simulink model "ControlOrientedModelsOfSeriesHybridElectricPowertrain"  (R2018b)
settings: Solver=VariableStepAuto  StartTime=0.0  StopTime=400  FixedStep=Tp  RelTol=1e-3
values from neighbouring files (symbols this model uses):
  R_wheel = 0.3    [data.mat]
  road =     [data.mat]
  StartPosition = 1600    [data.mat]
  V0 = 0    [data.mat]
undefined symbols (not defined in the file or in its folder): magnitude
libraries: simulink x6, simulink_extras x2, autolibshared x1
settings Model: SimulationMode=accelerator  Creator=piotr  LastModifiedBy=piotr
settings SolverCC: MaxConsecutiveMinStep=auto  ZeroCrossAlgorithm=Adaptive
settings OptimizationCC: EfficientMapNaN2IntZero=off
settings DebuggingCC: IgnoredZcDiagnostic=none  UnderSpecifiedDimensionMsg=warning
settings HardwareCC: TargetBitPerLong=64  TargetBitPerPointer=64  TargetBitPerSizeT=64  TargetBitPerPtrDiffT=64  TargetLongLongMode=on  TargetIntDivRoundTo=Zero  TargetEndianess=LittleEndian  TargetWordSize=64  TargetHWDeviceType=MATLAB Host  ProdEqTarget=off
settings CodeAppCC: MaxIdLength=128
settings GRTTargetCC: TargetLangStandard=C89/C90 (ANSI)  CombineOutputUpdateFcns=off  GRTInterface=on

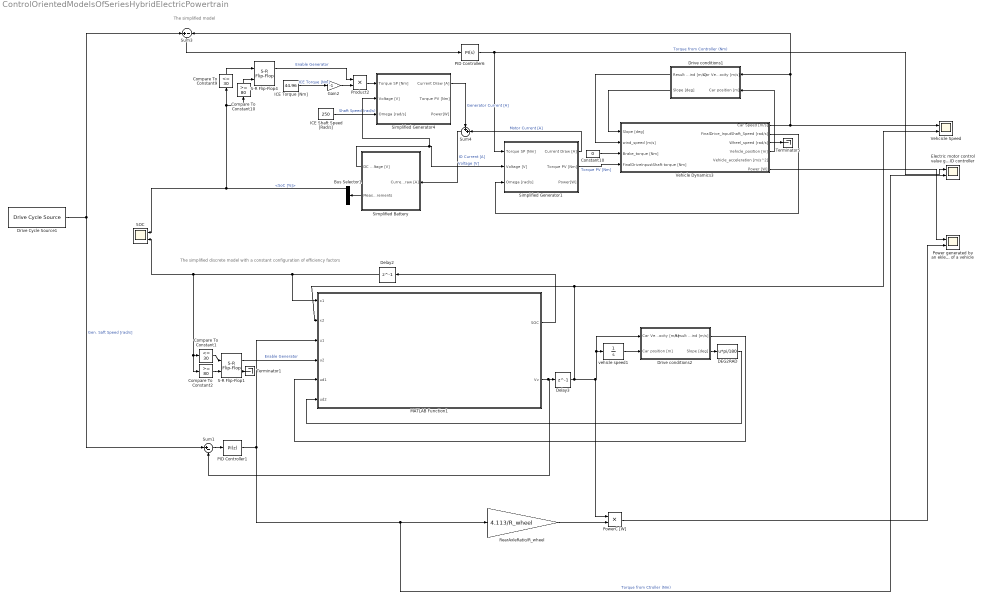
== system ControlOrientedModelsOfSeriesHybridElectricPowertrain ==
  note: The simplified discrete model with a constant configuration of efficiency factors
  note: The simplified model
  Bus Selector1 : BusSelector  OutputSignals=SoC [%],Power [W],IO Current [A]
  Compare To Constant1 : simulink/Logic and Bit Operations/Compare To Constant  relop=<=  const=30  OutDataTypeStr=boolean
  Compare To Constant10 : simulink/Logic and Bit Operations/Compare To Constant  relop=>=  const=80  OutDataTypeStr=boolean
  Compare To Constant2 : simulink/Logic and Bit Operations/Compare To Constant  relop=>=  const=80  OutDataTypeStr=boolean
  Compare To Constant9 : simulink/Logic and Bit Operations/Compare To Constant  relop=<=  const=30  OutDataTypeStr=boolean
  Constant10 : Constant  Value=0
  DEG2RAD : Fcn  Expr=u*pi/180
  Delay2 : Delay  DelayLength=1  InitialCondition=31  SampleTime=0.001
  Delay3 : Delay  DelayLength=1  InitialCondition=0  SampleTime=0.001
  Drive Cycle Source1 : autolibshared/Drive Cycle Source  cycleVar=FTP75  fileVar=cycleFTP75.mat  tfinal="2474  seconds"  cycleRepeat=off  outAccPort=off  outGearPort=off  gearList=No gear data  t_wot1=5  xdot_woto=0  xdot_wot1=30  t_wot2=20  xdot_wot2=0  t_wotend=30  srcUnit=m/s  outUnit=m/s  srcAccUnit=m/s/s  outAccUnit=m/s^2  dt=0  aMode=1
      settings: SourceProductName=Powertrain Blockset  SourceProductBaseCode=PW
  Drive conditions1 : Subsystem
  Drive conditions2 : Subsystem
  Electric motor control value generated by the PID controller : Scope  NumInputPorts=2
  Gain2 : Gain  Gain=-1
  ICE Shaft Speed [Rad/s] : Constant  Value=250
  ICE Torque [Nm] : Constant  Value=44.96
  MATLAB Function1 : MATLAB Function  TreatAsAtomicUnit=on
  PID Controller1 : simulink/Continuous/PID Controller  Controller=PI  Form=Parallel  TimeDomain=Discrete-time  SampleTime=0.001  IntegratorMethod=Forward Euler  FilterMethod=Forward Euler  ControllerParametersSource=internal  P=50  I=5  D=0  UseFilter=on  N=100  TunerSelectOption=Transfer Function Based (PID Tuner App)  InitialConditionSource=internal  InitialConditionForIntegrator=0  InitialConditionForFilter=0  DifferentiatorICPrevScaledInput=0  ExternalReset=none  TrackingMode=off  Kt=1  LimitOutput=off  UpperSaturationLimit=inf  LowerSaturationLimit=-inf  LinearizeAsGain=on  AntiWindupMode=none  Kb=1  POutMin=[]  POutMax=[]  IOutMin=[]  IOutMax=[]  DOutMin=[]  DOutMax=[]  NOutMin=[]  NOutMax=[]  SumOutMin=[]  SumOutMax=[]  SaturationOutMin=[]  SaturationOutMax=[]  PParamMin=[]  PParamMax=[]  IParamMin=[]  IParamMax=[]  DParamMin=[]  DParamMax=[]  NParamMin=[]  NParamMax=[]  KbParamMin=[]  KbParamMax=[]  KtParamMin=[]  KtParamMax=[]  KbOutMin=[]  KbOutMax=[]  KtOutMin=[]  KtOutMax=[]  IntegratorOutMin=[]  IntegratorOutMax=[]  FilterOutMin=[]  FilterOutMax=[]  SumI1OutMin=[]  SumI1OutMax=[]  SumI2OutMin=[]  SumI2OutMax=[]  SumI3OutMin=[]  SumI3OutMax=[]  SumI4OutMin=[]  SumI4OutMax=[]  SumDOutMin=[]  SumDOutMax=[]  DifferentiatorOutMin=[]  DifferentiatorOutMax=[]  FilterDiffOutCoefMin=[]  FilterDiffOutCoefMax=[]  ReciprocalOutMin=[]  ReciprocalOutMax=[]  SumDenOutMin=[]  SumDenOutMax=[]  SumNumOutMin=[]  SumNumOutMax=[]  DivideOutMin=[]  DivideOutMax=[]  IntegratorContinuousStateAttributes=''  IntegratorStateMustResolveToSignalObject=off  IntegratorRTWStateStorageClass=Auto  FilterContinuousStateAttributes=''  FilterStateMustResolveToSignalObject=off  FilterRTWStateStorageClass=Auto  ParallelPVariant=InternalParameters  IdealPVariant=Disabled  IVariant=InternalParameters  DVariant=Disabled  IntegratorVariant=Discrete  SatVariant=Disabled  AWVariant=Passthrough  PCopyVariant=Disabled  TRVariant=Disabled  FdbkBlocksVariant=Forward  IdealPFdbkVariant=Disabled  SatFdbkVariant=Disabled  DerivativeFilterVariant=Disabled  NVariant=Disabled  NCopyVariant=Disabled_SignalSpec  FilterICVariant=Disabled  IntegratorICVariant=InternalICs  ExternalResetVariant=Disabled  TRSumVariant=Passthrough  SumFdbkVariant=Disabled  SumVariant=Sum_PI
  PID Controller6 : simulink/Continuous/PID Controller  Controller=PI  Form=Parallel  TimeDomain=Continuous-time  SampleTime=-1  IntegratorMethod=Forward Euler  FilterMethod=Forward Euler  ControllerParametersSource=internal  P=50  I=5  D=0  UseFilter=on  N=100  TunerSelectOption=Transfer Function Based (PID Tuner App)  InitialConditionSource=internal  InitialConditionForIntegrator=0  InitialConditionForFilter=0  DifferentiatorICPrevScaledInput=0  ExternalReset=none  TrackingMode=off  Kt=1  LimitOutput=off  UpperSaturationLimit=inf  LowerSaturationLimit=-inf  LinearizeAsGain=on  AntiWindupMode=none  Kb=1  POutMin=[]  POutMax=[]  IOutMin=[]  IOutMax=[]  DOutMin=[]  DOutMax=[]  NOutMin=[]  NOutMax=[]  SumOutMin=[]  SumOutMax=[]  SaturationOutMin=[]  SaturationOutMax=[]  PParamMin=[]  PParamMax=[]  IParamMin=[]  IParamMax=[]  DParamMin=[]  DParamMax=[]  NParamMin=[]  NParamMax=[]  KbParamMin=[]  KbParamMax=[]  KtParamMin=[]  KtParamMax=[]  KbOutMin=[]  KbOutMax=[]  KtOutMin=[]  KtOutMax=[]  IntegratorOutMin=[]  IntegratorOutMax=[]  FilterOutMin=[]  FilterOutMax=[]  SumI1OutMin=[]  SumI1OutMax=[]  SumI2OutMin=[]  SumI2OutMax=[]  SumI3OutMin=[]  SumI3OutMax=[]  SumI4OutMin=[]  SumI4OutMax=[]  SumDOutMin=[]  SumDOutMax=[]  DifferentiatorOutMin=[]  DifferentiatorOutMax=[]  FilterDiffOutCoefMin=[]  FilterDiffOutCoefMax=[]  ReciprocalOutMin=[]  ReciprocalOutMax=[]  SumDenOutMin=[]  SumDenOutMax=[]  SumNumOutMin=[]  SumNumOutMax=[]  DivideOutMin=[]  DivideOutMax=[]  IntegratorContinuousStateAttributes=''  IntegratorStateMustResolveToSignalObject=off  IntegratorRTWStateStorageClass=Auto  FilterContinuousStateAttributes=''  FilterStateMustResolveToSignalObject=off  FilterRTWStateStorageClass=Auto  ParallelPVariant=InternalParameters  IdealPVariant=Disabled  IVariant=InternalParameters  DVariant=Disabled  IntegratorVariant=Continuous  SatVariant=Disabled  AWVariant=Passthrough  PCopyVariant=Disabled  TRVariant=Disabled  FdbkBlocksVariant=Forward  IdealPFdbkVariant=Disabled  SatFdbkVariant=Disabled  DerivativeFilterVariant=Disabled  NVariant=Disabled  NCopyVariant=Disabled_SignalSpec  FilterICVariant=Disabled  IntegratorICVariant=InternalICs  ExternalResetVariant=Disabled  TRSumVariant=Passthrough  SumFdbkVariant=Disabled  SumVariant=Sum_PI
  "Power generated by an eklectric motor driving the wheels of a vehicle " : Scope  NumInputPorts=2
  PowerC [W] : Product
  Product2 : Product
  RearAxleRatio/R_wheel : Gain  Gain=4.113/R_wheel
  S-R Flip-Flop1 : simulink_extras/Flip Flops/S-R Flip-Flop  initial_condition=0
  S-R Flip-Flop4 : simulink_extras/Flip Flops/S-R Flip-Flop  initial_condition=0
  "SOC " : Scope  NumInputPorts=2
  Simplified Battery : Subsystem  mask(Simple Battery with DC/DC converter){VIO=500, VBatt=200, CapBatt=7, Isoc=31, CHCoeff=75, DCoeff=90}
      mask prompts: VIO "DC Source Voltage I/O"; VBatt "DC Battery Inside Model Voltage"; CapBatt "Battery Capacity [Ah] Reffers to Battery Inside Model Voltage"; Isoc "Initial SOC [0-100%]"; CHCoeff "Charging Coefficient [0-100%]"; DCoeff "Draw Energy Coefficient [0-100%]"
  Simplified Generator1 : Subsystem  mask(Simplify Electric Motor/Generator){GCoeff=85, UCoeff=100}
      mask prompts: GCoeff "Generator performance [0-100%]"; UCoeff "Motor Performance [0-100%]"
      mask help: Block converts electric energy into mechanical energy. Torque set point is limited by torque vs speed table. Block calculates current draw and electric motor/generator torque within given radial speed. In Generator mode negative torque gives current.
  Simplified Generator4 : Subsystem  mask(Simplify Electric Motor/Generator){GCoeff=95, UCoeff=100}
      mask prompts: GCoeff "Generator performance [0-100%]"; UCoeff "Motor Performance [0-100%]"
      mask help: Block converts electric energy into mechanical energy. Torque set point is limited by torque vs speed table. Block calculates current draw and electric motor/generator torque within given radial speed. In Generator mode negative torque gives current.
  Sum1 : Sum  Inputs=|+-
  Sum3 : Sum  Inputs=+-
  Sum4 : Sum  Inputs=++|
  Terminator1 : Terminator
  Terminator5 : Terminator
  Vehcicle Speed : Scope  NumInputPorts=2
  Vehicle Dynamics3 : Subsystem
  vehicle speed1 : Integrator  InitialCondition=StartPosition  LimitOutput=on  LowerSaturationLimit=0  ZeroCross=off
  wires:
  MATLAB Function1/1(SOC) -> Delay2/1
  PID Controller1/1 -> Electric motor control value generated by the PID controller/2, RearAxleRatio/R_wheel/1, MATLAB Function1/3(u1)  "Torque from Ctroller (Nm)"
  S-R Flip-Flop1/2 -> Terminator1/1
  Compare To Constant1/1 -> S-R Flip-Flop1/1
  Sum1/1 -> PID Controller1/1
  Compare To Constant2/1 -> S-R Flip-Flop1/2
  Delay2/1 -> MATLAB Function1/1(x1), Compare To Constant2/1, Compare To Constant1/1, "SOC "/2
  Delay3/1 -> PowerC [W]/1, Drive conditions2/1(Car Velocity [m/s]), vehicle speed1/1, Vehcicle Speed/2, MATLAB Function1/2(x2)
  PID Controller6/1 -> Electric motor control value generated by the PID controller/1, Simplified Generator1/1(Torque SP [Nm])  "Torque from Controller (Nm)"
  Product2/1 -> Simplified Generator4/1(Torque SP [Nm])
  Simplified Battery/2(Measurements) -> Bus Selector1/1
  Drive Cycle Source1/1 -> Sum1/1, Sum3/1  "Gen. Saft Speed [rad/s]"
  Vehicle Dynamics3/1(Car Speed [m/s]) -> Drive conditions1/1(Car Velocity [m/s]), Sum3/2, Vehcicle Speed/1
  ICE Torque [Nm]/1 -> Gain2/1  "ICE Torque [Nm]"
  Simplified Generator1/1(Current Draw [A]) -> Sum4/2  "Motor Current [A]"
  Simplified Generator1/2(Torque PV [Nm]) -> Vehicle Dynamics3/4(FinalDriveInpustShaft torque [Nm])  "Torque PV [Nm]"
  Bus Selector1/1 -> "SOC "/1, Compare To Constant9/1, Compare To Constant10/1  "<SoC [%]>"
  Gain2/1 -> Product2/2
  Vehicle Dynamics3/2(FinalDrive_InputShaft_Speed [rad/s]) -> Simplified Generator1/3(Omega [rad/s])
  Sum4/1 -> Simplified Battery/1(Current Draw [A])  "IO Current [A]"
  S-R Flip-Flop4/1 -> Product2/1  "Enable Generator"
  Sum3/1 -> PID Controller6/1
  Constant10/1 -> Vehicle Dynamics3/3(Brake_torque [Nm])
  Simplified Battery/1(DC Output Voltage [V]) -> Simplified Generator1/2(Voltage [V]), Simplified Generator4/2(Voltage [V])  "Voltage [V]"
  Compare To Constant10/1 -> S-R Flip-Flop4/2
  Simplified Generator4/1(Current Draw [A]) -> Sum4/1  "Generator Current [A]"
  ICE Shaft Speed [Rad/s]/1 -> Simplified Generator4/3(Omega [rad/s])  "Shaft Speed (rad/s)"
  Vehicle Dynamics3/3(Wheel_speed [rad/s]) -> Terminator5/1
  Compare To Constant9/1 -> S-R Flip-Flop4/1
  RearAxleRatio/R_wheel/1 -> PowerC [W]/2
  S-R Flip-Flop1/1 -> MATLAB Function1/4(u2)  "Enable Generator"
  MATLAB Function1/2(Vv) -> Sum1/2, Delay3/1
  Vehicle Dynamics3/4(Vehicle_position [m]) -> Drive conditions1/2(Car position [m])
  Drive conditions1/1(Result Wind [m/s]) -> Vehicle Dynamics3/2(wind_speed [m/s])
  vehicle speed1/1 -> Drive conditions2/2(Car position [m])
  Drive conditions2/1(Result Wind [m/s]) -> MATLAB Function1/5(ud1)
  Drive conditions2/2(Slope [deg]) -> DEG2RAD/1
  Drive conditions1/2(Slope [deg]) -> Vehicle Dynamics3/1(Slope [deg])
  DEG2RAD/1 -> MATLAB Function1/6(ud2)
  Vehicle Dynamics3/6(Power [W]) -> "Power generated by an eklectric motor driving the wheels of a vehicle "/1
  PowerC [W]/1 -> "Power generated by an eklectric motor driving the wheels of a vehicle "/2

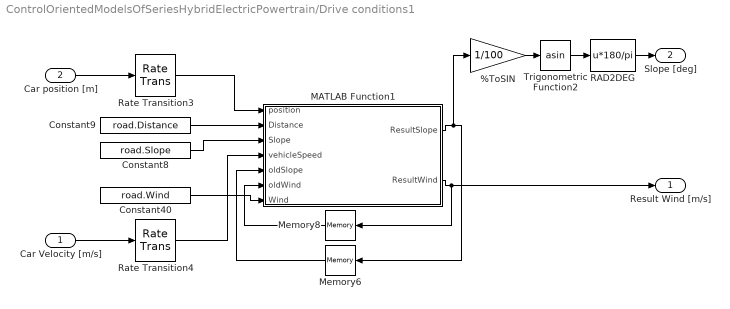
== system ControlOrientedModelsOfSeriesHybridElectricPowertrain/Drive conditions1 ==
  Car Velocity [m/s] : Inport
  Car position [m] : Inport  Port=2
  %ToSIN : Gain  Gain=1/100
  Constant40 : Constant  Value=road.Wind
  Constant8 : Constant  Value=road.Slope
  Constant9 : Constant  Value=road.Distance
  MATLAB Function1 : MATLAB Function  TreatAsAtomicUnit=on
  Memory6 : Memory  InheritSampleTime=on
  Memory8 : Memory  InheritSampleTime=on
  RAD2DEG : Fcn  Expr=u*180/pi
  Rate Transition3 : RateTransition  OutPortSampleTime=Ts_GPC
  Rate Transition4 : RateTransition  OutPortSampleTime=Ts_GPC
  Trigonometric Function2 : Trigonometry  Operator=asin
  Result Wind [m/s] : Outport
  Slope [deg] : Outport  Port=2
  wires:
  Constant40/1 -> MATLAB Function1/7(Wind)
  MATLAB Function1/1(ResultSlope) -> Memory6/1, %ToSIN/1
  Rate Transition3/1 -> MATLAB Function1/1(position)
  Memory8/1 -> MATLAB Function1/6(oldWind)
  Rate Transition4/1 -> MATLAB Function1/4(vehicleSpeed)
  Trigonometric Function2/1 -> RAD2DEG/1
  Constant9/1 -> MATLAB Function1/2(Distance)
  MATLAB Function1/2(ResultWind) -> Result Wind [m/s]/1, Memory8/1
  Memory6/1 -> MATLAB Function1/5(oldSlope)
  Constant8/1 -> MATLAB Function1/3(Slope)
  %ToSIN/1 -> Trigonometric Function2/1
  RAD2DEG/1 -> Slope [deg]/1
  Car Velocity [m/s]/1 -> Rate Transition4/1
  Car position [m]/1 -> Rate Transition3/1

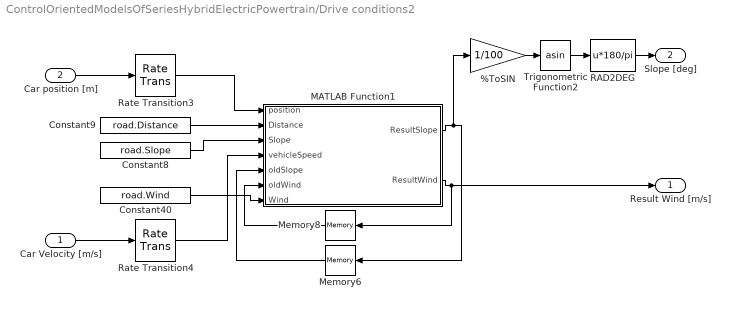
== system ControlOrientedModelsOfSeriesHybridElectricPowertrain/Drive conditions2 ==
  Car Velocity [m/s] : Inport
  Car position [m] : Inport  Port=2
  %ToSIN : Gain  Gain=1/100
  Constant40 : Constant  Value=road.Wind
  Constant8 : Constant  Value=road.Slope
  Constant9 : Constant  Value=road.Distance
  MATLAB Function1 : MATLAB Function  TreatAsAtomicUnit=on
  Memory6 : Memory  InheritSampleTime=on
  Memory8 : Memory  InheritSampleTime=on
  RAD2DEG : Fcn  Expr=u*180/pi
  Rate Transition3 : RateTransition  OutPortSampleTime=Ts_GPC
  Rate Transition4 : RateTransition  OutPortSampleTime=Ts_GPC
  Trigonometric Function2 : Trigonometry  Operator=asin
  Result Wind [m/s] : Outport
  Slope [deg] : Outport  Port=2
  wires:
  Constant40/1 -> MATLAB Function1/7(Wind)
  MATLAB Function1/1(ResultSlope) -> Memory6/1, %ToSIN/1
  Rate Transition3/1 -> MATLAB Function1/1(position)
  Memory8/1 -> MATLAB Function1/6(oldWind)
  Rate Transition4/1 -> MATLAB Function1/4(vehicleSpeed)
  Trigonometric Function2/1 -> RAD2DEG/1
  Constant9/1 -> MATLAB Function1/2(Distance)
  MATLAB Function1/2(ResultWind) -> Result Wind [m/s]/1, Memory8/1
  Memory6/1 -> MATLAB Function1/5(oldSlope)
  Constant8/1 -> MATLAB Function1/3(Slope)
  %ToSIN/1 -> Trigonometric Function2/1
  RAD2DEG/1 -> Slope [deg]/1
  Car Velocity [m/s]/1 -> Rate Transition4/1
  Car position [m]/1 -> Rate Transition3/1

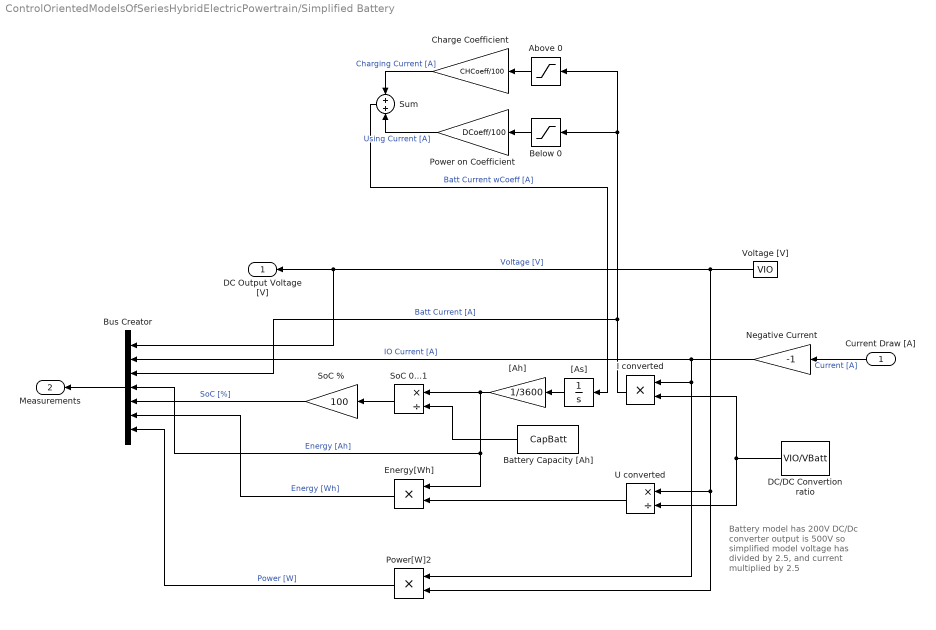
== system ControlOrientedModelsOfSeriesHybridElectricPowertrain/Simplified Battery ==
  note: Battery model has 200V DC/Dc converter output is 500V so simplified model voltage has divided by 2.5, and current multiplied by 2.5
  Current Draw [A] : Inport
  Above 0 : Saturate  UpperLimit=inf  LowerLimit=0
  Battery Capacity [Ah] : Constant  Value=CapBatt
  Below 0 : Saturate  UpperLimit=0  LowerLimit=-inf
  Bus Creator : BusCreator  Inputs=7
  Charge Coefficient : Gain  Gain=CHCoeff/100
  DC/DC Convertion ratio : Constant  Value=VIO/VBatt
  Energy[Wh] : Product
  I converted : Product  Inputs=**
  Negative Current : Gain  Gain=-1
  Power on Coefficient : Gain  Gain=DCoeff/100
  Power[W]2 : Product
  SoC % : Gain  Gain=100
  SoC 0...1 : Product  Inputs=*/
  Sum : Sum
  U converted : Product  Inputs=*/
  Voltage [V] : Constant  Value=VIO
  "[Ah]" : Gain  Gain=1/3600
  "[As]" : Integrator  InitialCondition=Isoc*CapBatt*3600/100
  DC Output Voltage [V] : Outport
  Measurements : Outport  Port=2
  wires:
  "[Ah]"/1 -> Bus Creator/4, Energy[Wh]/1, SoC 0...1/1  "Energy [Ah]"
  Voltage [V]/1 -> Bus Creator/1, DC Output Voltage [V]/1, Power[W]2/2, U converted/1  "Voltage [V]"
  Energy[Wh]/1 -> Bus Creator/6  "Energy [Wh]"
  Battery Capacity [Ah]/1 -> SoC 0...1/2
  I converted/1 -> Above 0/1, Below 0/1, Bus Creator/3  "Batt Current [A]"
  Current Draw [A]/1 -> Negative Current/1  "Current [A]"
  SoC 0...1/1 -> SoC %/1
  "[As]"/1 -> "[Ah]"/1
  SoC %/1 -> Bus Creator/5  "SoC [%]"
  Power[W]2/1 -> Bus Creator/7  "Power [W]"
  U converted/1 -> Energy[Wh]/2
  DC/DC Convertion ratio/1 -> U converted/2, I converted/2
  Negative Current/1 -> Power[W]2/1, I converted/1, Bus Creator/2  "IO Current [A]"
  Bus Creator/1 -> Measurements/1
  Below 0/1 -> Power on Coefficient/1
  Above 0/1 -> Charge Coefficient/1
  Power on Coefficient/1 -> Sum/2  "Using Current [A]"
  Charge Coefficient/1 -> Sum/1  "Charging Current [A]"
  Sum/1 -> "[As]"/1  "Batt Current wCoeff [A]"

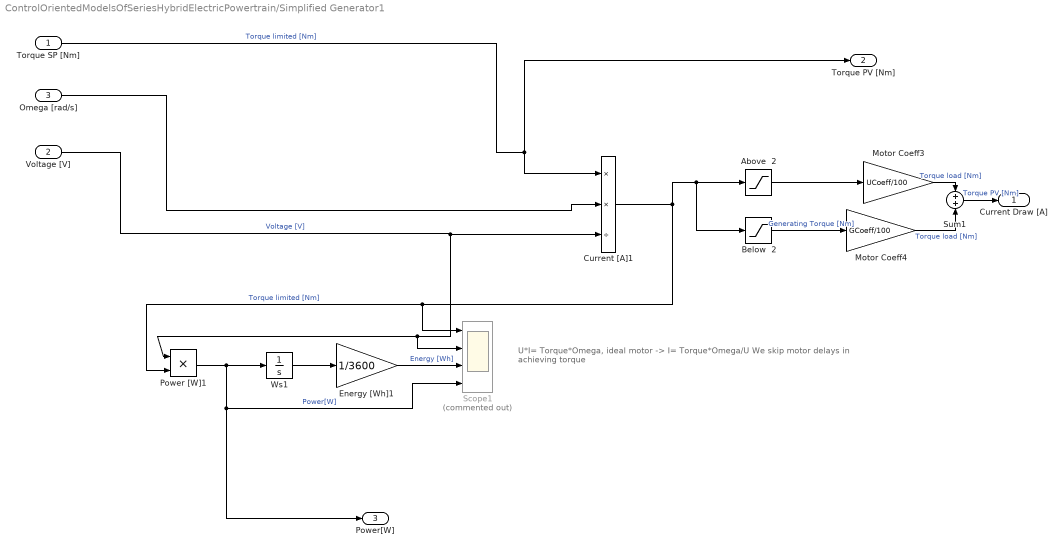
== system ControlOrientedModelsOfSeriesHybridElectricPowertrain/Simplified Generator1 ==
  note: U*I= Torque*Omega, ideal motor
      | -> I= Torque*Omega/U
      | We skip motor delays in achieving torque
  Torque SP [Nm] : Inport
  Voltage [V] : Inport  Port=2
  Omega [rad/s] : Inport  Port=3
  Above  2 : Saturate  UpperLimit=inf  LowerLimit=0
  Below  2 : Saturate  UpperLimit=0  LowerLimit=-inf
  Current [A]1 : Product  Inputs=**/
  Energy [Wh]1 : Gain  Gain=1/3600
  Motor Coeff3 : Gain  Gain=UCoeff/100
  Motor Coeff4 : Gain  Gain=GCoeff/100
  Power [W]1 : Product
  Scope1 : Scope  Commented=on  NumInputPorts=4
  Sum1 : Sum
  Ws1 : Integrator
  Current Draw [A] : Outport
  Torque PV [Nm] : Outport  Port=2
  Power[W] : Outport  Port=3
  wires:
  Ws1/1 -> Energy [Wh]1/1
  Power [W]1/1 -> Scope1/4, Power[W]/1, Ws1/1  "Power[W]"
  Voltage [V]/1 -> Power [W]1/1, Scope1/2, Current [A]1/3  "Voltage [V]"
  Energy [Wh]1/1 -> Scope1/3  "Energy [Wh]"
  Torque SP [Nm]/1 -> Torque PV [Nm]/1, Current [A]1/1  "Torque limited [Nm]"
  Omega [rad/s]/1 -> Current [A]1/2
  Below  2/1 -> Motor Coeff4/1  "Generating Torque [Nm]"
  Above  2/1 -> Motor Coeff3/1
  Current [A]1/1 -> Below  2/1, Above  2/1, Power [W]1/2, Scope1/1  "Torque limited [Nm]"
  Motor Coeff4/1 -> Sum1/2  "Torque load [Nm]"
  Motor Coeff3/1 -> Sum1/1  "Torque load [Nm]"
  Sum1/1 -> Current Draw [A]/1  "Torque PV [Nm]"

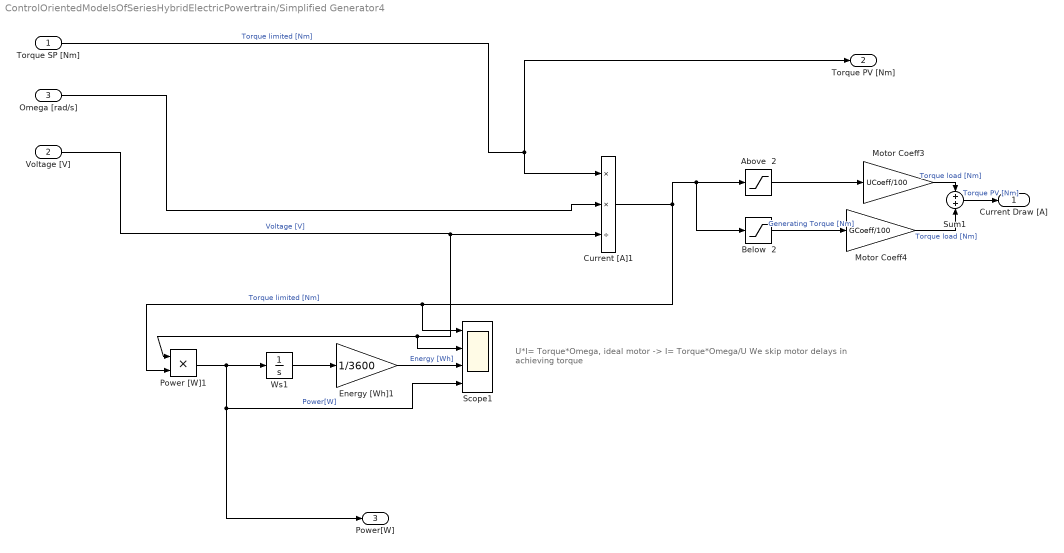
== system ControlOrientedModelsOfSeriesHybridElectricPowertrain/Simplified Generator4 ==
  note: U*I= Torque*Omega, ideal motor
      | -> I= Torque*Omega/U
      | We skip motor delays in achieving torque
  Torque SP [Nm] : Inport
  Voltage [V] : Inport  Port=2
  Omega [rad/s] : Inport  Port=3
  Above  2 : Saturate  UpperLimit=inf  LowerLimit=0
  Below  2 : Saturate  UpperLimit=0  LowerLimit=-inf
  Current [A]1 : Product  Inputs=**/
  Energy [Wh]1 : Gain  Gain=1/3600
  Motor Coeff3 : Gain  Gain=UCoeff/100
  Motor Coeff4 : Gain  Gain=GCoeff/100
  Power [W]1 : Product
  Scope1 : Scope  NumInputPorts=4
  Sum1 : Sum
  Ws1 : Integrator
  Current Draw [A] : Outport
  Torque PV [Nm] : Outport  Port=2
  Power[W] : Outport  Port=3
  wires:
  Ws1/1 -> Energy [Wh]1/1
  Power [W]1/1 -> Scope1/4, Power[W]/1, Ws1/1  "Power[W]"
  Voltage [V]/1 -> Power [W]1/1, Scope1/2, Current [A]1/3  "Voltage [V]"
  Energy [Wh]1/1 -> Scope1/3  "Energy [Wh]"
  Torque SP [Nm]/1 -> Torque PV [Nm]/1, Current [A]1/1  "Torque limited [Nm]"
  Omega [rad/s]/1 -> Current [A]1/2
  Below  2/1 -> Motor Coeff4/1  "Generating Torque [Nm]"
  Above  2/1 -> Motor Coeff3/1
  Current [A]1/1 -> Below  2/1, Above  2/1, Power [W]1/2, Scope1/1  "Torque limited [Nm]"
  Motor Coeff4/1 -> Sum1/2  "Torque load [Nm]"
  Motor Coeff3/1 -> Sum1/1  "Torque load [Nm]"
  Sum1/1 -> Current Draw [A]/1  "Torque PV [Nm]"

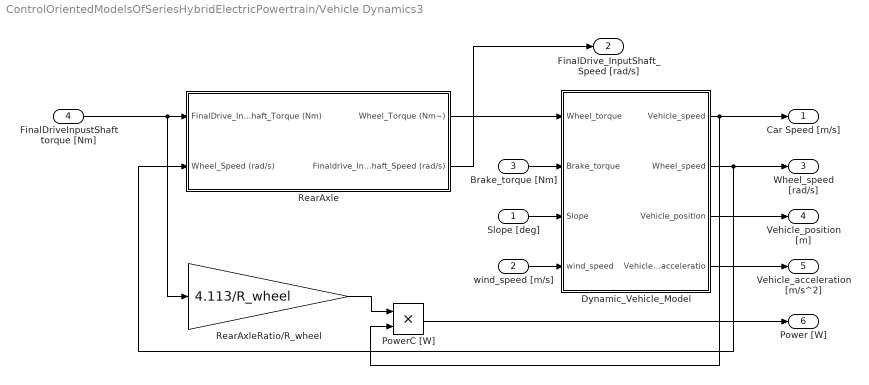
== system ControlOrientedModelsOfSeriesHybridElectricPowertrain/Vehicle Dynamics3 ==
  Slope [deg] : Inport
  wind_speed [m/s] : Inport  Port=2
  Brake_torque [Nm] : Inport  Port=3
  FinalDriveInpustShaft torque [Nm] : Inport  Port=4
  Dynamic_Vehicle_Model : Subsystem  mask(Vehicle Model){TotalVehicleMass=1085, GravitationalAcceleration=9.81, AirDensity=1.13, FrontalAreaOfVehicle=2.54, AirResistanceCoefficient=0.26, TotalNumberOfWheels=4, InertiaOfWheel=1.7, WheelRadius=0.3, DrivingResistanceCoefficient=0.015, StartPosition=StartPosition, V0=V0}
      mask prompts: TotalVehicleMass "TotalVehicle"; V0 "InitialSpeed"
      mask help:
      | Dynamic vehicle Model
      | Simple Model that considers
      | 1. Downhill slope force (down- and uphill)
      | 2. Driving rsistence force
      | 3. Airdynamic resistence force
      | 4. Inertia of wheels
      | 5. Inertia of vehicle mass
      |
      | Parameters :
      | TotalVehicleMass in [kg]
      | GravitationalAcceleration 9.81 [m/s^2] on earth
      | WheelRadius in [m]: center of rim to surface of tyre
      | TotalNumberOfWheels: total number of wheels included on a vehicle
      | InertiaOfWheels: rim and tyre for one wheel
      | DrivingResistanceCoefficient: 0.015 to 0.025 values from liertature, this is a tuning parameter
      | AirDensity - 1.15 [kg/m^3] - dependent on air temperature and air pressure
      | AirResistanceCoefficient - 0.45 dependend on vehicle type/size, speed etc.
      | FrontalAreaOfVehicle - 3.32 [m^2] dependent on vehicle type
      |
      | Inputs:
      | Wheel_torque [Nm]:  torque from rear axle
      | Brake_torque [Nm]: torque applied to the wheels by brake system
      | Wind_speed [m/s]: direction blowing against vehicle
      | Slope:  slope of road in degree-positive value -> uphill
      |
      | Output:
      | Wheel_speed [rpm]: revolutios per minute of wheels
      | Vehicle_acceleratio [m/s^2]: vehicle acceleratio
      | Vehicle_speed [m/s]: vehicle speed
      | Vehicle_position [m]: vehicle x position
  PowerC [W] : Product
  RearAxle : Subsystem  mask(Vehicle Model){RearAxleRatio=4.113, RearAxleEffeciency=0.97}
      mask help:
      | Rear axle model of a vehicle
      |
      | Axle input speed (rpm_at_gearbox)=Axle output speed (rpm_at_wheel)* RearAxleRatio
      | Axle output torque (wheel_torque)=Axle input troque (GearboxOutputTorque)* RearAxleRatio *RearAxleEffeciency
  RearAxleRatio/R_wheel : Gain  Gain=4.113/R_wheel
  Car Speed [m/s] : Outport
  FinalDrive_InputShaft_Speed [rad/s] : Outport  Port=2  InitialOutput=0
  Wheel_speed [rad/s] : Outport  Port=3
  Vehicle_position [m] : Outport  Port=4
  Vehicle_acceleration [m/s^2] : Outport  Port=5
  Power [W] : Outport  Port=6
  wires:
  Slope [deg]/1 -> Dynamic_Vehicle_Model/3(Slope)
  wind_speed [m/s]/1 -> Dynamic_Vehicle_Model/4(wind_speed)
  Dynamic_Vehicle_Model/2(Wheel_speed) -> Wheel_speed [rad/s]/1, RearAxle/2(Wheel_Speed (rad/s))
  Dynamic_Vehicle_Model/4(Vehicle_acceleratio) -> Vehicle_acceleration [m/s^2]/1
  Dynamic_Vehicle_Model/3(Vehicle_position) -> Vehicle_position [m]/1
  RearAxle/1(Wheel_Torque (Nm~)) -> Dynamic_Vehicle_Model/1(Wheel_torque)
  Brake_torque [Nm]/1 -> Dynamic_Vehicle_Model/2(Brake_torque)
  Dynamic_Vehicle_Model/1(Vehicle_speed) -> PowerC [W]/2, Car Speed [m/s]/1
  FinalDriveInpustShaft torque [Nm]/1 -> RearAxleRatio/R_wheel/1, RearAxle/1(FinalDrive_InputShaft_Torque (Nm))
  RearAxle/2(Finaldrive_InputShaft_Speed (rad/s)) -> FinalDrive_InputShaft_Speed [rad/s]/1
  RearAxleRatio/R_wheel/1 -> PowerC [W]/1
  PowerC [W]/1 -> Power [W]/1

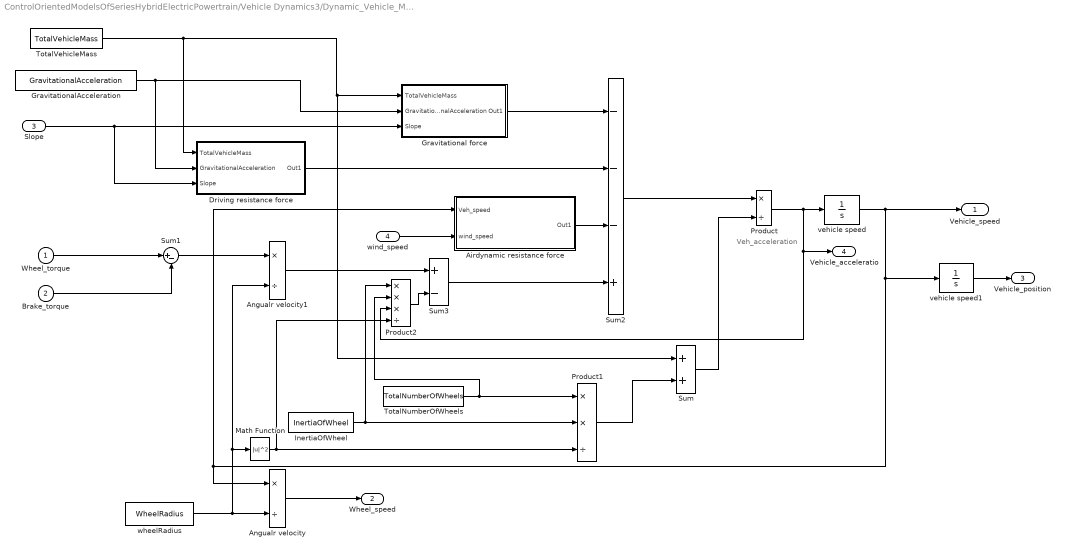
== system ControlOrientedModelsOfSeriesHybridElectricPowertrain/Vehicle Dynamics3/Dynamic_Vehicle_Model ==
  note: Veh_acceleration
  Wheel_torque : Inport
  Brake_torque : Inport  Port=2
  Slope : Inport  Port=3
  wind_speed : Inport  Port=4
  Airdynamic resistance force : Subsystem
  Angualr velocity : Product  Inputs=*/
  Angualr velocity1 : Product  Inputs=*/
  Driving resistance force : Subsystem
  Gravitational force : Subsystem
  GravitationalAcceleration : Constant  Value=GravitationalAcceleration
  InertiaOfWheel : Constant  Value=InertiaOfWheel
  Math Function : Math  Operator=magnitude^2  SaturateOnIntegerOverflow=on
  Product : Product  Inputs=*/  RndMeth=Zero
  Product1 : Product  Inputs=**/  RndMeth=Zero
  Product2 : Product  Inputs=***/  RndMeth=Zero
  Sum : Sum
  Sum1 : Sum  Inputs=|+-
  Sum2 : Sum  Inputs=---+  SaturateOnIntegerOverflow=on  InputSameDT=on  OutDataTypeStr=Inherit: Same as first input
  Sum3 : Sum  Inputs=+-
  TotalNumberOfWheels : Constant  Value=TotalNumberOfWheels
  TotalVehicleMass : Constant  Value=TotalVehicleMass
  vehicle speed : Integrator  InitialCondition=V0  LimitOutput=on  ZeroCross=off
  vehicle speed1 : Integrator  InitialCondition=StartPosition  LimitOutput=on  LowerSaturationLimit=0  ZeroCross=off
  wheelRadius : Constant  Value=WheelRadius
  Vehicle_speed : Outport  InitialOutput=0
  Wheel_speed : Outport  Port=2
  Vehicle_position : Outport  Port=3
  Vehicle_acceleratio : Outport  Port=4
  wires:
  Sum2/1 -> Product/1
  Product/1 -> Product2/3, Vehicle_acceleratio/1, vehicle speed/1
  Sum/1 -> Product/2
  Wheel_torque/1 -> Sum1/1
  Sum1/1 -> Angualr velocity1/1
  wind_speed/1 -> Airdynamic resistance force/2(wind_speed)
  TotalNumberOfWheels/1 -> Product2/2, Product1/1
  Angualr velocity/1 -> Wheel_speed/1
  wheelRadius/1 -> Angualr velocity/2, Angualr velocity1/2, Math Function/1
  Product1/1 -> Sum/2
  Brake_torque/1 -> Sum1/2
  Gravitational force/1(Out1) -> Sum2/1
  vehicle speed/1 -> Vehicle_speed/1, vehicle speed1/1, Airdynamic resistance force/1(Veh_speed), Angualr velocity/1
  Angualr velocity1/1 -> Sum3/1
  InertiaOfWheel/1 -> Product2/1, Product1/2
  TotalVehicleMass/1 -> Driving resistance force/1(TotalVehicleMass), Sum/1, Gravitational force/1(TotalVehicleMass)
  GravitationalAcceleration/1 -> Driving resistance force/2(GravitationalAcceleration), Gravitational force/2(GravitationalAcceleration)
  Slope/1 -> Gravitational force/3(Slope), Driving resistance force/3(Slope)
  Driving resistance force/1(Out1) -> Sum2/2
  Airdynamic resistance force/1(Out1) -> Sum2/3
  vehicle speed1/1 -> Vehicle_position/1
  Sum3/1 -> Sum2/4
  Product2/1 -> Sum3/2
  Math Function/1 -> Product2/4, Product1/3

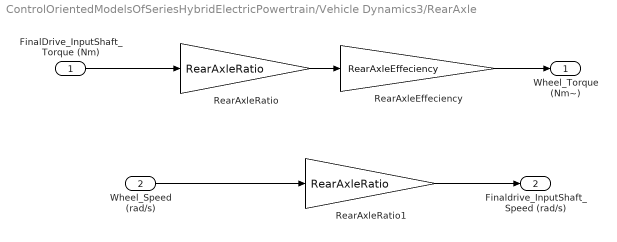
== system ControlOrientedModelsOfSeriesHybridElectricPowertrain/Vehicle Dynamics3/RearAxle ==
  FinalDrive_InputShaft_Torque (Nm) : Inport
  Wheel_Speed (rad/s) : Inport  Port=2
  RearAxleEffeciency : Gain  Gain=RearAxleEffeciency  SaturateOnIntegerOverflow=on  OutDataTypeStr=Inherit: Same as input  ParamDataTypeStr=Inherit: Same as input
  RearAxleRatio : Gain  Gain=RearAxleRatio  SaturateOnIntegerOverflow=on  OutDataTypeStr=Inherit: Same as input  ParamDataTypeStr=Inherit: Same as input
  RearAxleRatio1 : Gain  Gain=RearAxleRatio  SaturateOnIntegerOverflow=on  OutDataTypeStr=Inherit: Same as input  ParamDataTypeStr=Inherit: Same as input
  Wheel_Torque (Nm~) : Outport
  Finaldrive_InputShaft_Speed (rad/s) : Outport  Port=2
  wires:
  FinalDrive_InputShaft_Torque (Nm)/1 -> RearAxleRatio/1
  RearAxleRatio1/1 -> Finaldrive_InputShaft_Speed (rad/s)/1
  RearAxleRatio/1 -> RearAxleEffeciency/1
  Wheel_Speed (rad/s)/1 -> RearAxleRatio1/1
  RearAxleEffeciency/1 -> Wheel_Torque (Nm~)/1

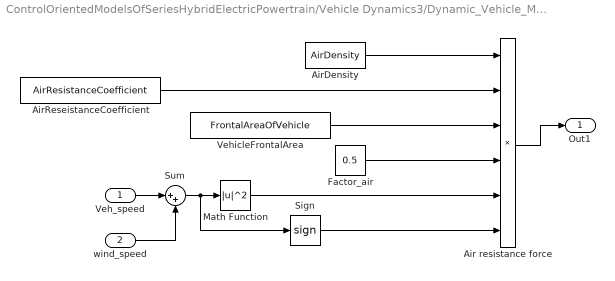
== system ControlOrientedModelsOfSeriesHybridElectricPowertrain/Vehicle Dynamics3/Dynamic_Vehicle_Model/Airdynamic resistance force ==
  Veh_speed : Inport
  wind_speed : Inport  Port=2
  Air resistance force : Product  Inputs=6
  AirDensity : Constant  Value=AirDensity
  AirReseistanceCoefficient : Constant  Value=AirResistanceCoefficient
  Factor_air : Constant  Value=0.5
  Math Function : Math  Operator=magnitude^2  SaturateOnIntegerOverflow=on
  Sign : Signum
  Sum : Sum  Inputs=|++
  VehicleFrontalArea : Constant  Value=FrontalAreaOfVehicle
  Out1 : Outport
  wires:
  Air resistance force/1 -> Out1/1
  wind_speed/1 -> Sum/2
  Veh_speed/1 -> Sum/1
  Sum/1 -> Sign/1, Math Function/1
  Math Function/1 -> Air resistance force/5
  Factor_air/1 -> Air resistance force/4
  VehicleFrontalArea/1 -> Air resistance force/3
  AirReseistanceCoefficient/1 -> Air resistance force/2
  AirDensity/1 -> Air resistance force/1
  Sign/1 -> Air resistance force/6

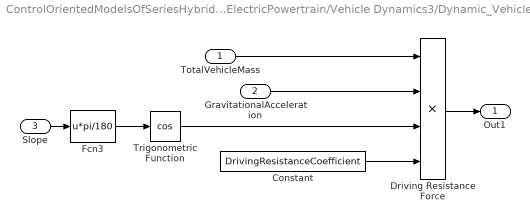
== system ControlOrientedModelsOfSeriesHybridElectricPowertrain/Vehicle Dynamics3/Dynamic_Vehicle_Model/Driving resistance force ==
  TotalVehicleMass : Inport
  GravitationalAcceleration : Inport  Port=2
  Slope : Inport  Port=3
  Constant : Constant  Value=DrivingResistanceCoefficient
  Driving Resistance Force : Product  Inputs=4
  Fcn3 : Fcn  Expr=u*pi/180
  Trigonometric Function : Trigonometry  Operator=cos
  Out1 : Outport
  wires:
  Driving Resistance Force/1 -> Out1/1
  Constant/1 -> Driving Resistance Force/4
  TotalVehicleMass/1 -> Driving Resistance Force/1
  GravitationalAcceleration/1 -> Driving Resistance Force/2
  Slope/1 -> Fcn3/1
  Fcn3/1 -> Trigonometric Function/1
  Trigonometric Function/1 -> Driving Resistance Force/3

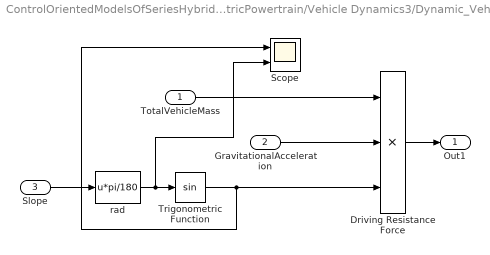
== system ControlOrientedModelsOfSeriesHybridElectricPowertrain/Vehicle Dynamics3/Dynamic_Vehicle_Model/Gravitational force ==
  TotalVehicleMass : Inport
  GravitationalAcceleration : Inport  Port=2
  Slope : Inport  Port=3
  Driving Resistance Force : Product  Inputs=3
  Scope : Scope  NumInputPorts=2
  Trigonometric Function : Trigonometry
  rad : Fcn  Expr=u*pi/180
  Out1 : Outport
  wires:
  Driving Resistance Force/1 -> Out1/1
  TotalVehicleMass/1 -> Driving Resistance Force/1
  GravitationalAcceleration/1 -> Driving Resistance Force/2
  Slope/1 -> rad/1
  rad/1 -> Scope/2, Trigonometric Function/1
  Trigonometric Function/1 -> Scope/1, Driving Resistance Force/3

== matlab function ControlOrientedModelsOfSeriesHybridElectricPowertrain/MATLAB Function1 ==
  data: x1 input size=1; x2 input size=1; u1 input size=1; u2 input size=1; SOC output size=1; ud1 input size=1; ud2 input size=1; Vv output size=1
function [SOC,Vv] = SimplifiedDiscreteModelWithAConstantConfigurationOfEfficiencyFactors(x1,x2,u1, u2,ud1,ud2)
SOC = (5339*u2)/31200000 + x1 - (457*u1*x2)/2080000000;
 
 
Vv = (1196883*u1)/104450000000 + x2 - (5747679*cos(ud2))/41780000000 - (1915893*sin(ud2))/208900000 - (1679067*(ud1 + x2)^2)/5222500000000 ;
    %SOC x1
    %Vv x2
    %TMSP -u1
    %Eg - u2
    %vw - ud1
    %theta - ud2
  
end

== matlab function ControlOrientedModelsOfSeriesHybridElectricPowertrain/Drive conditions1/MATLAB Function1 ==
  data: position input; ResultSlope output; Distance input; Slope input; vehicleSpeed input; oldSlope input; oldWind input; Wind input; ResultWind output
function [ResultSlope, ResultWind] = PPmap(position,Distance,Slope, vehicleSpeed,oldSlope,oldWind,Wind)

% Autor     : Paweł & Piotr
% Date      : March 2021
if vehicleSpeed>0.1
p=-inf;
i=0;
DistanceSize=size(Distance,1);

while p<position && i<DistanceSize
    i=i+1;
    p=Distance(i);
end

i=i-1;

ResultSlope= Slope(i)+((Slope(i+1)-Slope(i))/(Distance(i+1)-Distance(i)))*(position-Distance(i));
ResultWind= (Wind(i)+((Wind(i+1)-Wind(i))/(Distance(i+1)-Distance(i)))*(position-Distance(i)));
else
ResultSlope= oldSlope;
ResultWind=oldWind;
end
end

== matlab function ControlOrientedModelsOfSeriesHybridElectricPowertrain/Drive conditions2/MATLAB Function1 ==
  data: position input; ResultSlope output; Distance input; Slope input; vehicleSpeed input; oldSlope input; oldWind input; Wind input; ResultWind output
function [ResultSlope, ResultWind] = PPmap(position,Distance,Slope, vehicleSpeed,oldSlope,oldWind,Wind)

% Autor     : Paweł & Piotr
% Date      : March 2021
if vehicleSpeed>0.1
p=-inf;
i=0;
DistanceSize=size(Distance,1);

while p<position && i<DistanceSize
    i=i+1;
    p=Distance(i);
end

i=i-1;

ResultSlope= Slope(i)+((Slope(i+1)-Slope(i))/(Distance(i+1)-Distance(i)))*(position-Distance(i));
ResultWind= (Wind(i)+((Wind(i+1)-Wind(i))/(Distance(i+1)-Distance(i)))*(position-Distance(i)));
else
ResultSlope= oldSlope;
ResultWind=oldWind;
end
end
